simulink model "untitled"  (R2021b)
settings: Solver=FixedStepAuto  StartTime=0.0  StopTime=10.0  FixedStep=0.02  RelTol=1e-3
settings Model: Creator=GW00216231  LastModifiedBy=GW00216231

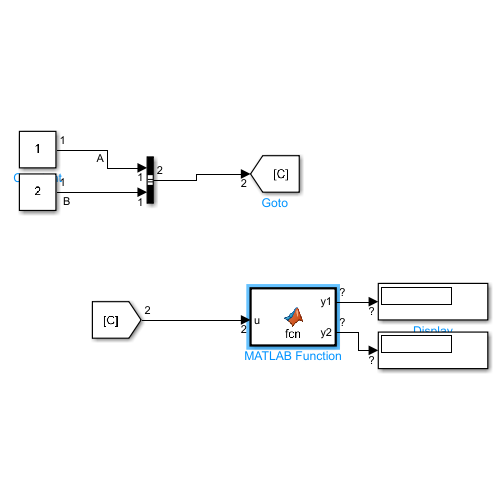
[thumbnail: Simulink's stored preview of the top-level diagram]
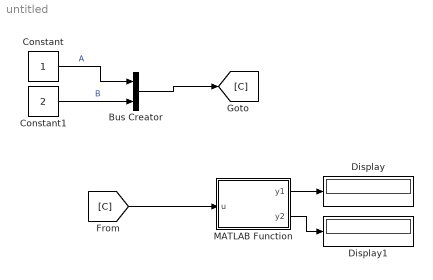
== system untitled ==
  Bus Creator : BusCreator  Inputs=2
  Constant : Constant
  Constant1 : Constant  Value=2
  Display : Display
  Display1 : Display
  MATLAB Function : MATLAB Function  TreatAsAtomicUnit=on
  wires:
  Constant/1 -> Bus Creator/1  "A"
  Constant1/1 -> Bus Creator/2  "B"
  Bus Creator/1 -> [C]
  [C] -> MATLAB Function/1(u)
  MATLAB Function/1(y1) -> Display/1
  MATLAB Function/2(y2) -> Display1/1

== matlab function untitled/MATLAB Function ==
  data: u input; y1 output; y2 output
function [y1,y2]= fcn(u)
y1 = u(1);
y2 = u(2);
end
